simulink model "Phase_reversal"  (R2022b)
settings: Solver=VariableStepAuto  StartTime=0.0  StopTime=10.0  RelTol=1e-3
libraries: spsControlledVoltageSourceLib x3, spsCurrentMeasurementLib x3, spsSeriesRLCBranchLib x3, spsSeriesRLCLoadLib x3, spsThreePhaseProgrammableGeneratorLib x3, simulink x2, spsGroundLib x2, spsThreePhaseProgrammableVoltageSourceLib x1, spsThreePhaseVIMeasurementLib x1, spsThreePhaseSourceLib x1, spsVoltageMeasurementLib x1, sps_lib x1
settings Model: Creator=E0660158  LastModifiedBy=E0660158

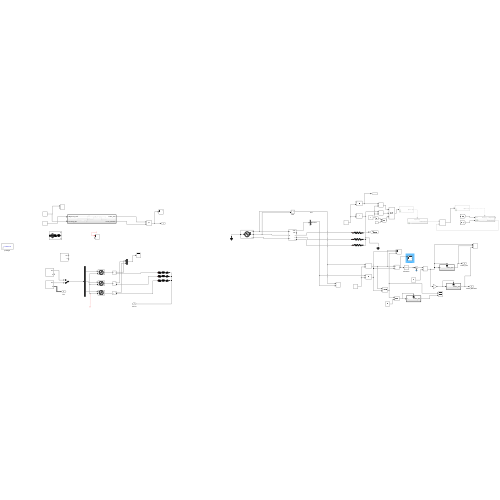
[thumbnail: Simulink's stored preview of the top-level diagram]
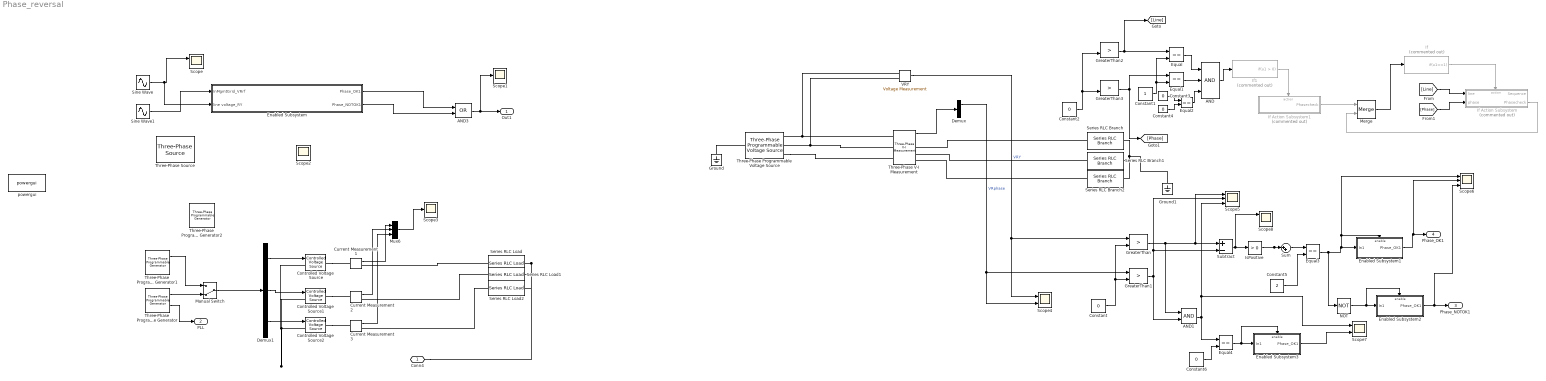
== system Phase_reversal ==
  AND : Logic  Inputs=3  AllPortsSameDT=off  OutDataTypeStr=boolean
  AND1 : Logic  AllPortsSameDT=off  OutDataTypeStr=boolean
  AND3 : Logic  Operator=OR  AllPortsSameDT=off  OutDataTypeStr=boolean
  Constant{,2..4,6} (5 alike) : Constant  Value=0
  Constant1 : Constant
  Constant5 : Constant  Value=2
  Controlled Voltage Source : spsControlledVoltageSourceLib/Controlled Voltage Source  Initialize=off  Source_Type=AC  Amplitude=0  Phase=0  Frequency=0  Measurements=None
  Controlled Voltage Source1 : spsControlledVoltageSourceLib/Controlled Voltage Source  Initialize=off  Source_Type=AC  Amplitude=0  Phase=0  Frequency=0  Measurements=None
  Controlled Voltage Source2 : spsControlledVoltageSourceLib/Controlled Voltage Source  Initialize=off  Source_Type=AC  Amplitude=0  Phase=0  Frequency=0  Measurements=None
  Current Measurement1 : spsCurrentMeasurementLib/Current Measurement  PhasorSimulation=off  OutputType=Complex  PSBequivalent=0
  Current Measurement2 : spsCurrentMeasurementLib/Current Measurement  PhasorSimulation=off  OutputType=Complex  PSBequivalent=0
  Current Measurement3 : spsCurrentMeasurementLib/Current Measurement  PhasorSimulation=off  OutputType=Complex  PSBequivalent=0
  Demux : Demux  Outputs=3
  Demux1 : Demux  Outputs=3
  Enabled Subsystem : Subsystem  TreatAsAtomicUnit=on
  Enabled Subsystem1 : Subsystem  TreatAsAtomicUnit=on
  Enabled Subsystem2 : Subsystem  TreatAsAtomicUnit=on
  Enabled Subsystem3 : Subsystem  TreatAsAtomicUnit=on
  Equal{,1..4} (5 alike) : RelationalOperator  Operator===  OutDataTypeStr=boolean  RndMeth=Simplest  InputSameDT=off
  GreaterThan{,1..3} (4 alike) : RelationalOperator  Operator=>  OutDataTypeStr=boolean  RndMeth=Simplest  InputSameDT=off
  Ground : spsGroundLib/Ground  LConnTagsString=a
  Ground1 : spsGroundLib/Ground  LConnTagsString=a
  If : If  Commented=on  IfExpression=u1==1  ShowElse=off
  If Action Subsystem : Subsystem  Commented=on  TreatAsAtomicUnit=on
  If Action Subsystem1 : Subsystem  Commented=on  TreatAsAtomicUnit=on
  If1 : If  Commented=on  ShowElse=off
  IsPositive : simulink/Logic and Bit Operations/Compare To Zero  relop=>  OutDataTypeStr=boolean
      settings: LibrarySourceBlock=|
      | simulink/Quick Insert/Logic and Bit
      | Operations/IsPositive
  Manual Switch : ManualSwitch  CurrentSetting=0
  Merge : Merge
  Mux6 : Mux  Inputs=3
  NOT : Logic  Operator=NOT  IconShape=distinctive  AllPortsSameDT=off  OutDataTypeStr=boolean
  Scope{,2,4,7} (4 alike) : Scope  NumInputPorts=2
  Scope1 : Scope
  Scope3 : Scope
  Scope5 : Scope  NumInputPorts=3
  Scope6 : Scope  NumInputPorts=3
  Scope8 : Scope  NumInputPorts=3
  Series RLC Branch : spsSeriesRLCBranchLib/Series RLC Branch  LConnTagsString=__new0  RConnTagsString=__new0  BranchType=R  Resistance=1  Inductance=1e-3  SetiL0=off  InitialCurrent=0  Capacitance=1e-6  Setx0=off  InitialVoltage=0  Measurements=None
  Series RLC Branch1 : spsSeriesRLCBranchLib/Series RLC Branch  LConnTagsString=__new0  RConnTagsString=__new0  BranchType=R  Resistance=1  Inductance=1e-3  SetiL0=off  InitialCurrent=0  Capacitance=1e-6  Setx0=off  InitialVoltage=0  Measurements=None
  Series RLC Branch2 : spsSeriesRLCBranchLib/Series RLC Branch  LConnTagsString=__new0  RConnTagsString=__new0  BranchType=R  Resistance=1  Inductance=1e-3  SetiL0=off  InitialCurrent=0  Capacitance=1e-6  Setx0=off  InitialVoltage=0  Measurements=None
  Series RLC Load : spsSeriesRLCLoadLib/Series RLC Load  LConnTagsString=a  RConnTagsString=__new0  NominalVoltage=240  NominalFrequency=50  ActivePower=10e3  InductivePower=100  CapacitivePower=100  Setx0=off  InitialVoltage=0  SetiL0=off  InitialCurrent=0  Measurements=None  LoadType=constant Z
  Series RLC Load1 : spsSeriesRLCLoadLib/Series RLC Load  LConnTagsString=a  RConnTagsString=__new0  NominalVoltage=240  NominalFrequency=50  ActivePower=10e3  InductivePower=100  CapacitivePower=100  Setx0=off  InitialVoltage=0  SetiL0=off  InitialCurrent=0  Measurements=None  LoadType=constant Z
  Series RLC Load2 : spsSeriesRLCLoadLib/Series RLC Load  LConnTagsString=a  RConnTagsString=__new0  NominalVoltage=240  NominalFrequency=50  ActivePower=10e3  InductivePower=100  CapacitivePower=100  Setx0=off  InitialVoltage=0  SetiL0=off  InitialCurrent=0  Measurements=None  LoadType=constant Z
  Sine Wave : Sin  Amplitude=10  Frequency=314
  Sine Wave1 : Sin  Amplitude=10  Frequency=314  Phase=30*pi/180
  Subtract : Sum  Inputs=+-
  Sum : Sum  Inputs=|++
  Three-Phase Programmable Generator : spsThreePhaseProgrammableGeneratorLib/Three-Phase Programmable Generator  Par_Vps=[240*1.414*1, 0, 50]  VariationEntity=None  VariationType=Ramp  VariationStep=-0.5  VariationRate=1/0.3  VariationMag=0.3  VariationFreq=2  Par_Timing_Variation="[0.9  1.2]"  SinglePhase=on  Yampli=[1 0.2 1.2 1.0]  Xtime=[0 0.1 0.15 0.2]  HarmonicGeneration=off  Par_HarmoA="[3  5  -25 0]"  Par_HarmoB="[5  10  35  2]"  Par_Timing_Harmo="[ 0.05  99]"  Ts=0
      settings: LibrarySourceBlock=|
      | sps_lib/Sources/Signal Generator Sources/Three-Phase
      | Programmable
      | Generator
  Three-Phase Programmable Generator1 : spsThreePhaseProgrammableGeneratorLib/Three-Phase Programmable Generator  Par_Vps=[240*1.414*1, 0, 52]  VariationEntity=None  VariationType=Ramp  VariationStep=-0.5  VariationRate=-240*1.414*1*0.3/0.3  VariationMag=0.3  VariationFreq=2  Par_Timing_Variation="[0.25  0.55]"  SinglePhase=on  Yampli=[1 0.2 1.2 1.0]  Xtime=[0 0.1 0.15 0.2]  HarmonicGeneration=off  Par_HarmoA="[3  5  -25 0]"  Par_HarmoB="[5  10  35  2]"  Par_Timing_Harmo="[ 0.05  99]"  Ts=0
      settings: LibrarySourceBlock=|
      | sps_lib/Sources/Signal Generator Sources/Three-Phase
      | Programmable
      | Generator
  Three-Phase Programmable Generator2 : spsThreePhaseProgrammableGeneratorLib/Three-Phase Programmable Generator  Par_Vps=[100, 0, 60]  VariationEntity=None  VariationType=Ramp  VariationStep=-0.5  VariationRate=10  VariationMag=0.3  VariationFreq=2  Par_Timing_Variation="[0.2  1.2]"  SinglePhase=on  Yampli=[1 0.2 1.2 1.0]  Xtime=[0 0.1 0.15 0.2]  HarmonicGeneration=off  Par_HarmoA="[3  5  -25 0]"  Par_HarmoB="[5  10  35  2]"  Par_Timing_Harmo="[ 0.05  99]"  Ts=0
      settings: LibrarySourceBlock=|
      | sps_lib/Sources/Signal Generator Sources/Three-Phase
      | Programmable
      | Generator
  Three-Phase Programmable Voltage Source : spsThreePhaseProgrammableVoltageSourceLib/Three-Phase Programmable Voltage Source  PositiveSequence="[400  0 50]"  VariationEntity=None  VariationType=Table of time-amplitude pairs  VariationTypeAlt=Step  VariationStep=0.5  VariationRate=10  VariationMagnitude=0.3  VariationFrequency=2  VariationTiming=[1 2]  VariationPhaseA=off  Amplitudes=[1 0.8 1.2 1.0]  TimeValues=[0 0.1 0.15 0.2]  HarmonicGeneration=off  HarmonicA=[3 0.2 -25 0]  HarmonicB=[2 0.15 35 2]  Timing="[0.05  3]"  BusType=swing  Pref=0  Qref=0  Qmin=-inf  Qmax=inf
  Three-Phase V-I Measurement : spsThreePhaseVIMeasurementLib/Three-Phase V-I Measurement  VoltageMeasurement=phase-to-ground  SetLabelV=off  LabelV=Vabc  Vpu=off  VpuLL=off  CurrentMeasurement=yes  SetLabelI=off  LabelI=Iabc  Ipu=off  Pbase=100e6  Vbase=500e3  OutputType=Complex  PhasorSimulation=off  PSBequivalent=0
  Three-Phase Source : spsThreePhaseSourceLib/Three-Phase Source  InternalConnection=Yg  VoltagePhases=off  Voltage=25e3  PhaseAngle=0  Voltage_phases=[25e3 25e3 25e3]/sqrt(3)  PhaseAngles_phases=[0 -120 +120]  Frequency=60  NonIdealSource=on  SpecifyImpedance=off  Resistance=0.8929  Inductance=16.58e-3  ShortCircuitLevel=100e6  BaseVoltage=25e3  XRratio=7  BusType=swing  Pref=10e3  Qref=0  Prefabc=[10e3, 10e3, 10e3]  Qrefabc=[0, 0, 0]  Qmin=-inf  Qmax=inf
  VRY : spsVoltageMeasurementLib/Voltage Measurement  PhasorSimulation=off  OutputType=Complex  PSBequivalent=0
  powergui : sps_lib/powergui  Priority=1  SimulationMode=Continuous  SampleTime=50e-6  frequency=60  Iterations=50  frequencyindice=50  Pbase=100e6  ErrMax=1e-4  UnitsV=kV  UnitsW=MW  buscounter=0  FunctionMessages=off  echomessages=off  EnableUseOfTLC=off  CurrentSourceSwitches=off  DisableSnubberDevices=off  DisableRonSwitches=off  DisableVfSwitches=off  DisplayEquations=off  AutomaticDiscreteSolvers=off  SolverType=Tustin/Backward Euler (TBE)  Interpol=off  ExternalGateDelay=off  methode=off  Ts=100  x0status=blocks  SPID=on  SwTol=0  HookPort=off  NonlinearTolerance=1e-4  nMaxIteration=100  ContinueOnMaxIteration=off  RestoreLinks=warning  ResistiveCurrentMeasurement=off  Frange=[0:2:500]  Ylog=off  Xlog=on  ShowGrid=off  save=off  variable=ZData  structure=0  ZoomFFT=off  StartTime=0.0  cycles=1  DisplayStyle=1  fundamental=60  FreqAxis=off  MaxFrequency=1000  frequencyindicesteady=1  RmsSteady=1  display=off
  Conn4 : PMIOPort  Side=Left
  Out1 : Outport
  PLL : Outport  Port=2  VectorParamsAs1DForOutWhenUnconnected=off
  Phase_NOTOK1 : Outport  Port=3
  Phase_OK1 : Outport  Port=4
  wires:
  Enabled Subsystem/2(Phase_NOTOK1) -> AND3/2
  Sine Wave/1 -> Enabled Subsystem/2(line voltage_RY), Scope/1
  Enabled Subsystem/1(Phase_OK1) -> AND3/1
  AND3/1 -> Scope1/1, Out1/1
  ? -> Scope2/1
  Three-Phase Programmable Generator/1 -> Manual Switch/2
  Manual Switch/1 -> Demux1/1
  Current Measurement2/1 -> Mux6/2
  Three-Phase Programmable Generator1/1 -> Manual Switch/1
  Demux1/2 -> Controlled Voltage Source1/1
  Demux1/3 -> Controlled Voltage Source2/1
  Demux1/1 -> Controlled Voltage Source/1
  Current Measurement1/1 -> Mux6/1
  Three-Phase Programmable Generator/2 -> PLL/1
  Current Measurement3/1 -> Mux6/3
  Mux6/1 -> Scope3/1
  Sine Wave1/1 -> Enabled Subsystem/1(InMgmtGrid_VRrf)
  Three-Phase V-I Measurement/1 -> Demux/1
  Demux/1 -> GreaterThan1/1, Scope4/2  "VRphase"
  VRY/1 -> GreaterThan/1, Scope4/1  "VRY"
  GreaterThan/1 -> Scope5/1, Subtract/1, AND1/1
  Constant/1 -> GreaterThan1/2, GreaterThan/2
  Subtract/1 -> Scope8/1, IsPositive/1
  Enabled Subsystem2/1(Phase_OK1) -> Scope6/3, Phase_NOTOK1/1
  Constant1/1 -> Equal/2, Equal1/2
  Equal/1 -> AND/1
  Equal1/1 -> AND/2
  Constant2/1 -> GreaterThan3/2, GreaterThan2/2
  GreaterThan3/1 -> [Phase], Equal1/1
  If/1 -> If Action Subsystem/Action
  GreaterThan2/1 -> [Line], Equal/1
  [Line] -> If Action Subsystem/1(line)
  [Phase] -> If Action Subsystem/2(phase)
  AND/1 -> If1/1
  If1/1 -> If Action Subsystem1/Action
  If Action Subsystem1/1(Phasecheck) -> Merge/1
  If Action Subsystem/2(Phasecheck) -> Merge/2
  Merge/1 -> If/1
  Constant3/1 -> Equal2/1
  Constant4/1 -> Equal2/2
  Equal2/1 -> AND/3
  Enabled Subsystem1/1(Phase_OK1) -> Scope6/2, Phase_OK1/1
  NOT/1 -> Enabled Subsystem2/Enable, Enabled Subsystem2/1(In1)
  IsPositive/1 -> Sum/2, Sum/1
  Sum/1 -> Equal3/1
  Constant5/1 -> Equal3/2
  Equal3/1 -> NOT/1, Enabled Subsystem1/Enable, Scope6/1, Enabled Subsystem1/1(In1)
  AND1/1 -> Scope5/3, Scope7/1, Equal4/1
  Equal4/1 -> Enabled Subsystem3/Enable, Enabled Subsystem3/1(In1)
  Constant6/1 -> Equal4/2
  Enabled Subsystem3/1(Phase_OK1) -> Scope7/2
  GreaterThan1/1 -> AND1/2, Subtract/2, Scope5/2
  connections:
  Controlled Voltage Source2/LConn1 -- Controlled Voltage Source/LConn1 -- Controlled Voltage Source1/LConn1
  Controlled Voltage Source1/RConn1 -- Current Measurement2/LConn1
  Controlled Voltage Source/RConn1 -- Current Measurement1/LConn1
  Controlled Voltage Source2/RConn1 -- Current Measurement3/LConn1
  Series RLC Load/RConn1 -- Series RLC Load2/RConn1 -- Conn4/RConn1 -- Series RLC Load1/RConn1
  Series RLC Load1/LConn1 -- Current Measurement2/RConn1
  Series RLC Load2/LConn1 -- Current Measurement3/RConn1
  Series RLC Load/LConn1 -- Current Measurement1/RConn1
  VRY/LConn1 -- Three-Phase Programmable Voltage Source/RConn1 -- Three-Phase V-I Measurement/LConn1
  VRY/LConn2 -- Three-Phase Programmable Voltage Source/RConn2 -- Three-Phase V-I Measurement/LConn2
  Three-Phase Programmable Voltage Source/RConn3 -- Three-Phase V-I Measurement/LConn3
  Ground/LConn1 -- Three-Phase Programmable Voltage Source/LConn1
  Series RLC Branch/LConn1 -- Three-Phase V-I Measurement/RConn1
  Series RLC Branch1/LConn1 -- Three-Phase V-I Measurement/RConn2
  Series RLC Branch2/LConn1 -- Three-Phase V-I Measurement/RConn3
  Series RLC Branch/RConn1 -- Series RLC Branch1/RConn1 -- Series RLC Branch2/RConn1 -- Ground1/LConn1

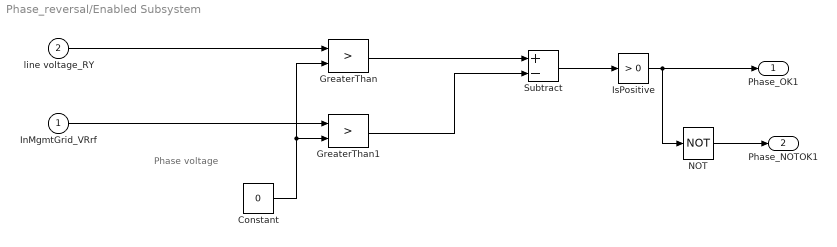
== system Phase_reversal/Enabled Subsystem ==
  note: Phase voltage
  InMgmtGrid_VRrf : Inport
  line voltage_RY : Inport  Port=2
  Constant : Constant  Value=0
  GreaterThan : RelationalOperator  Operator=>  OutDataTypeStr=boolean  RndMeth=Simplest  InputSameDT=off
  GreaterThan1 : RelationalOperator  Operator=>  OutDataTypeStr=boolean  RndMeth=Simplest  InputSameDT=off
  IsPositive : simulink/Logic and Bit Operations/Compare To Zero  relop=>  OutDataTypeStr=boolean
      settings: LibrarySourceBlock=|
      | simulink/Quick Insert/Logic and Bit
      | Operations/IsPositive
  NOT : Logic  Operator=NOT  IconShape=distinctive  AllPortsSameDT=off  OutDataTypeStr=boolean
  Subtract : Sum  Inputs=+-
  Phase_OK1 : Outport
  Phase_NOTOK1 : Outport  Port=2
  wires:
  NOT/1 -> Phase_NOTOK1/1
  GreaterThan/1 -> Subtract/1
  IsPositive/1 -> NOT/1, Phase_OK1/1
  GreaterThan1/1 -> Subtract/2
  Subtract/1 -> IsPositive/1
  Constant/1 -> GreaterThan1/2, GreaterThan/2
  line voltage_RY/1 -> GreaterThan/1
  InMgmtGrid_VRrf/1 -> GreaterThan1/1

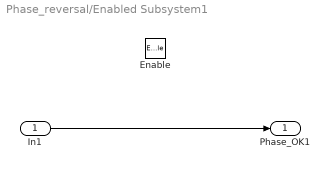
== system Phase_reversal/Enabled Subsystem1 ==
  In1 : Inport
  Enable : EnablePort
  Phase_OK1 : Outport
  wires:
  In1/1 -> Phase_OK1/1

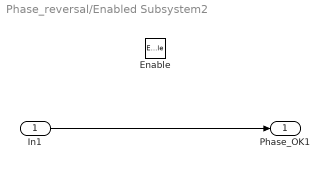
== system Phase_reversal/Enabled Subsystem2 ==
  In1 : Inport
  Enable : EnablePort
  Phase_OK1 : Outport
  wires:
  In1/1 -> Phase_OK1/1

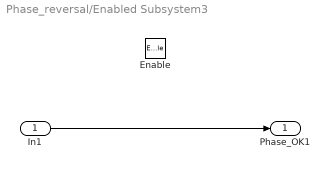
== system Phase_reversal/Enabled Subsystem3 ==
  In1 : Inport
  Enable : EnablePort
  Phase_OK1 : Outport
  wires:
  In1/1 -> Phase_OK1/1

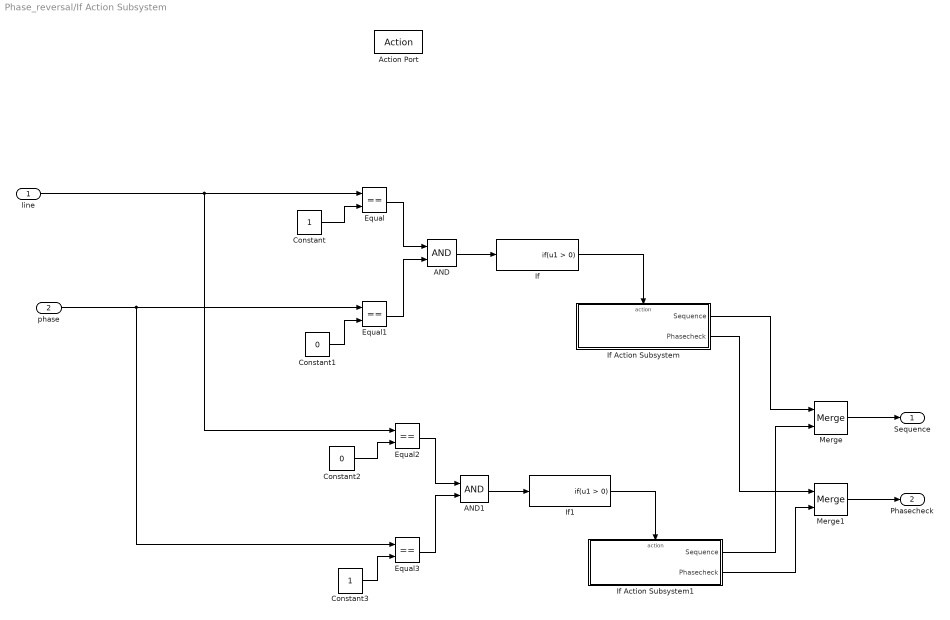
== system Phase_reversal/If Action Subsystem ==
  line : Inport
  phase : Inport  Port=2
  Action Port : ActionPort  ActionPortLabel=if(u1==1)
  AND : Logic  AllPortsSameDT=off  OutDataTypeStr=boolean
  AND1 : Logic  AllPortsSameDT=off  OutDataTypeStr=boolean
  Constant : Constant
  Constant1 : Constant  Value=0
  Constant2 : Constant  Value=0
  Constant3 : Constant
  Equal{,1..3} (4 alike) : RelationalOperator  Operator===  OutDataTypeStr=boolean  RndMeth=Simplest  InputSameDT=off
  If : If  ShowElse=off
  If Action Subsystem : Subsystem  TreatAsAtomicUnit=on
  If Action Subsystem1 : Subsystem  TreatAsAtomicUnit=on
  If1 : If  ShowElse=off
  Merge : Merge
  Merge1 : Merge
  Sequence : Outport
  Phasecheck : Outport  Port=2
  wires:
  line/1 -> Equal2/1, Equal/1
  Constant/1 -> Equal/2
  Constant1/1 -> Equal1/2
  Equal1/1 -> AND/2
  Equal/1 -> AND/1
  AND/1 -> If/1
  If/1 -> If Action Subsystem/Action
  If1/1 -> If Action Subsystem1/Action
  AND1/1 -> If1/1
  Equal2/1 -> AND1/1
  Equal3/1 -> AND1/2
  Constant3/1 -> Equal3/2
  phase/1 -> Equal3/1, Equal1/1
  Constant2/1 -> Equal2/2
  If Action Subsystem/1(Sequence) -> Merge/1
  If Action Subsystem1/1(Sequence) -> Merge/2
  Merge/1 -> Sequence/1
  If Action Subsystem/2(Phasecheck) -> Merge1/1
  If Action Subsystem1/2(Phasecheck) -> Merge1/2
  Merge1/1 -> Phasecheck/1

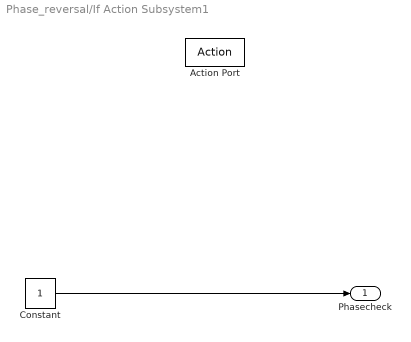
== system Phase_reversal/If Action Subsystem1 ==
  Action Port : ActionPort  ActionPortLabel=if(u1 > 0)
  Constant : Constant
  Phasecheck : Outport
  wires:
  Constant/1 -> Phasecheck/1

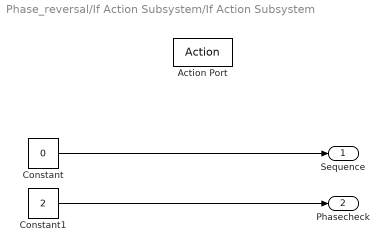
== system Phase_reversal/If Action Subsystem/If Action Subsystem ==
  Action Port : ActionPort  ActionPortLabel=if(u1 > 0)
  Constant : Constant  Value=0
  Constant1 : Constant  Value=2
  Sequence : Outport
  Phasecheck : Outport  Port=2
  wires:
  Constant/1 -> Sequence/1
  Constant1/1 -> Phasecheck/1

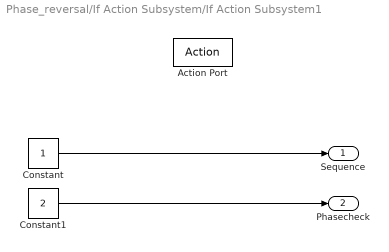
== system Phase_reversal/If Action Subsystem/If Action Subsystem1 ==
  Action Port : ActionPort  ActionPortLabel=if(u1 > 0)
  Constant : Constant
  Constant1 : Constant  Value=2
  Sequence : Outport
  Phasecheck : Outport  Port=2
  wires:
  Constant1/1 -> Phasecheck/1
  Constant/1 -> Sequence/1
